simulink model "sim3"  (R2022b)
settings: Solver=VariableStepAuto  StartTime=0.0  StopTime=100  RelTol=1e-3
values from neighbouring files (symbols this model uses):
  A_int = [A zeros(4,1); zeros(1,5)]    [main.m]
  B_int = [B; 0 0]    [main.m]
  C_int = eye(5)    [main.m]
  D_int = zeros(5,2)    [main.m]
  Klqr = lqr(A_int,B_int,Q,R)    [main.m]
  prek_sys_lqr = pinv([k_sys_lqr(1,1), k_sys_lqr(1,2);k_sys_lqr(5,1), k_sys_lqr(5,2)])    [main.m]
settings Model: Creator=augusto  LastModifiedBy=augusto

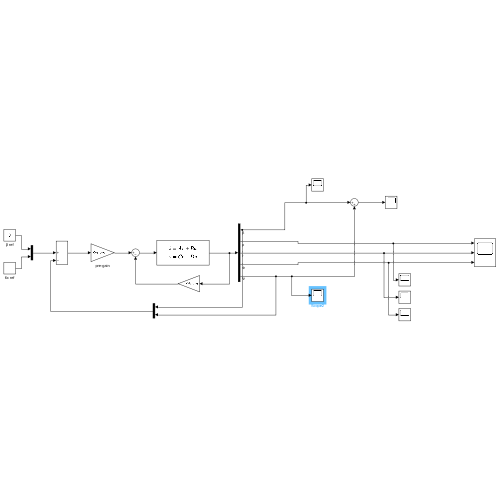
[thumbnail: Simulink's stored preview of the top-level diagram]
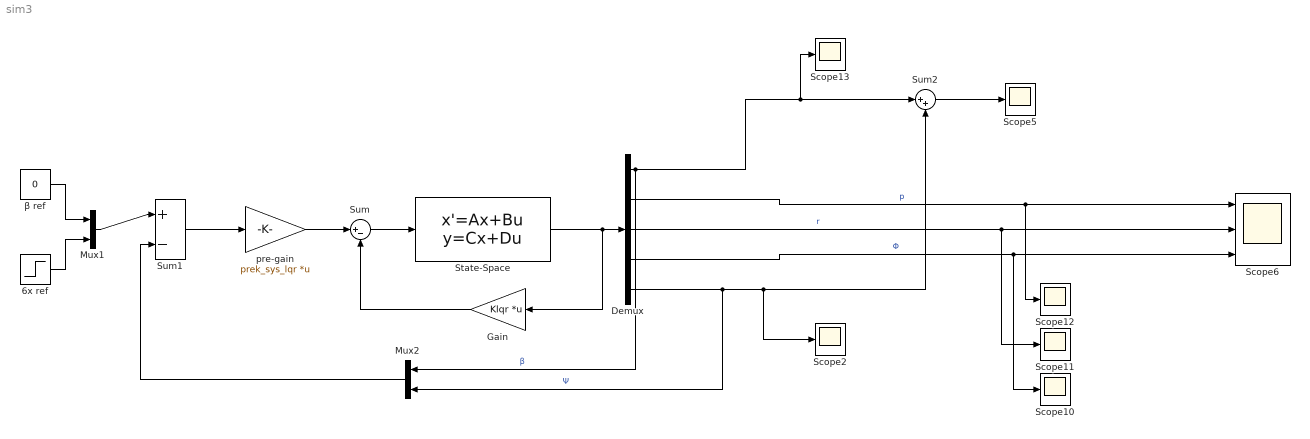
== system sim3 ==
  6x ref : Step  Time=deg2rad(60)  SampleTime=0
  Demux : Demux  Outputs=5
  Gain : Gain  Gain=Klqr  Multiplication=Matrix(K*u) (u vector)
  Mux1 : Mux  Inputs=2
  Mux2 : Mux  Inputs=2
  Scope{2,5,10..13} (6 alike) : Scope
  Scope6 : Scope  NumInputPorts=3
  State-Space : StateSpace  A=A_int  B=B_int  C=C_int  D=D_int  InitialCondition=0
  Sum : Sum  Inputs=|+-
  Sum1 : Sum  Inputs=|+-
  Sum2 : Sum  Inputs=|++
  pre-gain : Gain  Gain=prek_sys_lqr  Multiplication=Matrix(K*u) (u vector)
  β ref : Constant  Value=0
  wires:
  State-Space/1 -> Gain/1, Demux/1
  Demux/1 -> Mux2/1, Scope13/1, Sum2/1  "β"
  Sum/1 -> State-Space/1
  Gain/1 -> Sum/2
  Demux/5 -> Mux2/2, Sum2/2, Scope2/1  "Ψ"
  β ref/1 -> Mux1/1
  6x ref/1 -> Mux1/2
  Sum2/1 -> Scope5/1
  Sum1/1 -> pre-gain/1
  pre-gain/1 -> Sum/1
  Demux/3 -> Scope11/1, Scope6/2  "r"
  Demux/2 -> Scope12/1, Scope6/1  "p"
  Demux/4 -> Scope10/1, Scope6/3  "Φ"
  Mux1/1 -> Sum1/1
  Mux2/1 -> Sum1/2
